simulink model "Drv"  (R2020b)
settings: configuration reference "gen_config" (kept outside this file)
undefined symbols (not defined in the file): Bdy_lenRadiusWheel_C, Bdy_mEquivalentJ_C, Bdy_mVeh_C, Drv_kmh2gradtqDriver_C, Drv_kmh2tqDriver_C, kph2mps
libraries: simulink x2
settings Model: DataDictionary=Hybrid_vehicle.sldd  SimulationMode=accelerator  Creator=Georg  LastModifiedBy=jy
settings ConfigSetRef: SourceName=gen_config

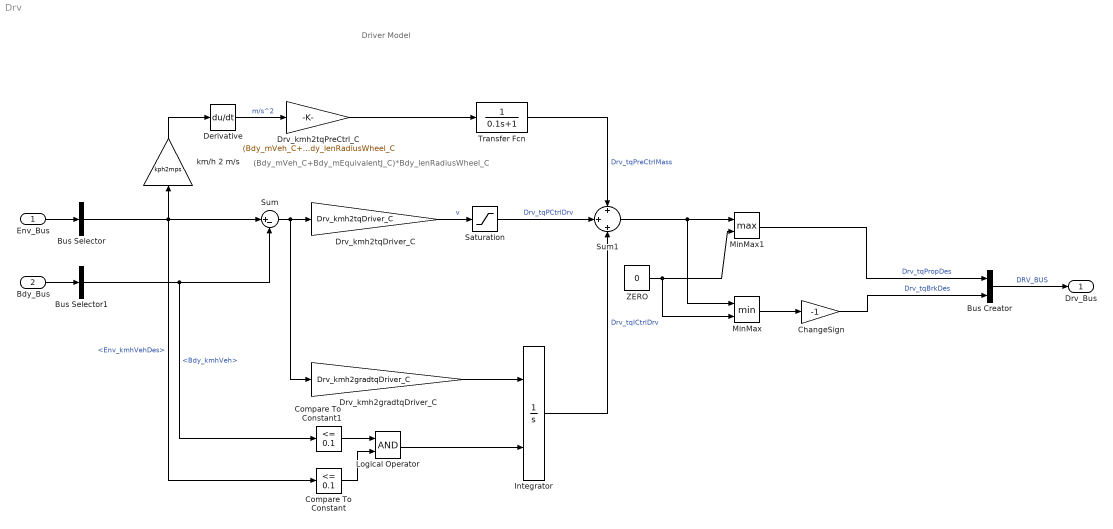
== system Drv ==
  note: Driver Model
  note: (Bdy_mVeh_C+Bdy_mEquivalentJ_C)*Bdy_lenRadiusWheel_C
  Env_Bus : Inport  OutDataTypeStr=Bus: ENV_BUS
  Bdy_Bus : Inport  Port=2  OutDataTypeStr=Bus: BDY_BUS
  Bus Creator : BusCreator  Inputs=2  OutDataTypeStr=Bus: DRV_BUS  NonVirtualBus=on
  Bus Selector : BusSelector  OutputSignals=Env_kmhVehDes
  Bus Selector1 : BusSelector  OutputSignals=Bdy_kmhVeh
  ChangeSign : Gain  Gain=-1
  Compare To Constant : simulink/Logic and Bit Operations/Compare To Constant  relop=<=  const=0.1  OutDataTypeStr=boolean
  Compare To Constant1 : simulink/Logic and Bit Operations/Compare To Constant  relop=<=  const=0.1  OutDataTypeStr=boolean
  Derivative : Derivative  CoefficientInTFapproximation=0.1
  Drv_kmh2gradtqDriver_C : Gain  Gain=Drv_kmh2gradtqDriver_C
  Drv_kmh2tqDriver_C : Gain  Gain=Drv_kmh2tqDriver_C
  Drv_kmh2tqPreCtrl_C : Gain  Gain=(Bdy_mVeh_C+Bdy_mEquivalentJ_C)*Bdy_lenRadiusWheel_C
  Integrator : Integrator  ExternalReset=level  InitialCondition=-10  LimitOutput=on  UpperSaturationLimit=1000  LowerSaturationLimit=-1000
  Logical Operator : Logic  AllPortsSameDT=off  OutDataTypeStr=boolean
  MinMax : MinMax  Inputs=2
  MinMax1 : MinMax  Function=max  Inputs=2
  Saturation : Saturate  UpperLimit=1000  LowerLimit=-1000
  Sum : Sum  Inputs=|+-
  Sum1 : Sum  Inputs=+|+|+
  Transfer Fcn : TransferFcn  Denominator=[0.1 1]
  ZERO : Constant  Value=0
  km/h 2 m/s : Gain  Gain=kph2mps
  Drv_Bus : Outport  OutDataTypeStr=Bus: DRV_BUS  VectorParamsAs1DForOutWhenUnconnected=off  BusOutputAsStruct=on
  wires:
  MinMax/1 -> ChangeSign/1
  Saturation/1 -> Sum1/2  "Drv_tqPCtrlDrv"
  Compare To Constant/1 -> Logical Operator/2
  Compare To Constant1/1 -> Logical Operator/1
  Logical Operator/1 -> Integrator/2
  MinMax1/1 -> Bus Creator/1  "Drv_tqPropDes"
  Drv_kmh2tqPreCtrl_C/1 -> Transfer Fcn/1
  Env_Bus/1 -> Bus Selector/1
  Sum1/1 -> MinMax/1, MinMax1/1
  km/h 2 m/s/1 -> Derivative/1
  Drv_kmh2tqDriver_C/1 -> Saturation/1  "v"
  ZERO/1 -> MinMax1/2, MinMax/2
  Bus Selector1/1 -> Compare To Constant1/1, Sum/2  "<Bdy_kmhVeh>"
  Bus Creator/1 -> Drv_Bus/1  "DRV_BUS"
  Drv_kmh2gradtqDriver_C/1 -> Integrator/1
  Transfer Fcn/1 -> Sum1/1  "Drv_tqPreCtrlMass"
  Bdy_Bus/1 -> Bus Selector1/1
  Derivative/1 -> Drv_kmh2tqPreCtrl_C/1  "m/s^2"
  Integrator/1 -> Sum1/3  "Drv_tqICtrlDrv"
  Bus Selector/1 -> km/h 2 m/s/1, Sum/1, Compare To Constant/1  "<Env_kmhVehDes>"
  Sum/1 -> Drv_kmh2tqDriver_C/1, Drv_kmh2gradtqDriver_C/1
  ChangeSign/1 -> Bus Creator/2  "Drv_tqBrkDes"
